simulink model "deadReckoning_VEX"  (R2017a)
settings: Solver=FixedStepAuto  StartTime=0.0  StopTime=inf  FixedStep=Ts  RelTol=1e-3  EnableMultiTasking=on
InitFcn:
  | robotParameters;
values from neighbouring files (symbols this model uses):
  ticksPerRot = 627.2    [robotParameters.m]
  Ts = 0.01    [robotParameters.m]
  wheelR = 0.052    [robotParameters.m]
undefined symbols (not defined in the file or in its folder): motorIp, motorSp
libraries: vexarmcortexlib x4, mobileRoboticsTrainingLib x1
settings Model: ExtModeTrigDuration=25  Creator=sseshadr  LastModifiedBy=shiremat
settings OptimizationCC: MaxStackSize=64
settings DebuggingCC: ParameterTunabilityLossMsg=error
settings HardwareCC: ProdBitPerPointer=32  ProdBitPerSizeT=32  ProdBitPerPtrDiffT=32  ProdLargestAtomicInteger=Long  ProdLargestAtomicFloat=Double  ProdWordSize=32  ProdHWDeviceType=ARM Compatible->ARM Cortex
settings SFSimCC: MATLABDynamicMemAlloc=off
settings RTWCC: SystemTargetFile=ert.tlc  HardwareBoard=ARM Cortex-based VEX Microcontroller  TLCOptions="-aInlineSetEventsForThisBaseRateFcn=TLC_FALSE -aSuppressMultiTaskScheduler=TLC_FALSE  -aRateBasedStepFcn=0"  TemplateMakefile=ert_default_tmf  Description=Embedded Coder  GenerateReport=on  Toolchain=GNU Tools for VEX ARM Cortex  IncludeHyperlinkInReport=on  LaunchReport=on  GenerateTraceInfo=on  GenerateTraceReport=on  GenerateTraceReportSl=on  GenerateTraceReportSf=on  GenerateTraceReportEml=on
settings CodeAppCC: ForceParamTrailComments=on  IgnoreCustomStorageClasses=off  OperatorAnnotations=on  SimulinkDataObjDesc=on  SFDataObjDesc=on  MATLABFcnDesc=on  InsertBlockDesc=on  MATLABSourceComments=on
settings ERTTargetCC: MultiwordLength=2048

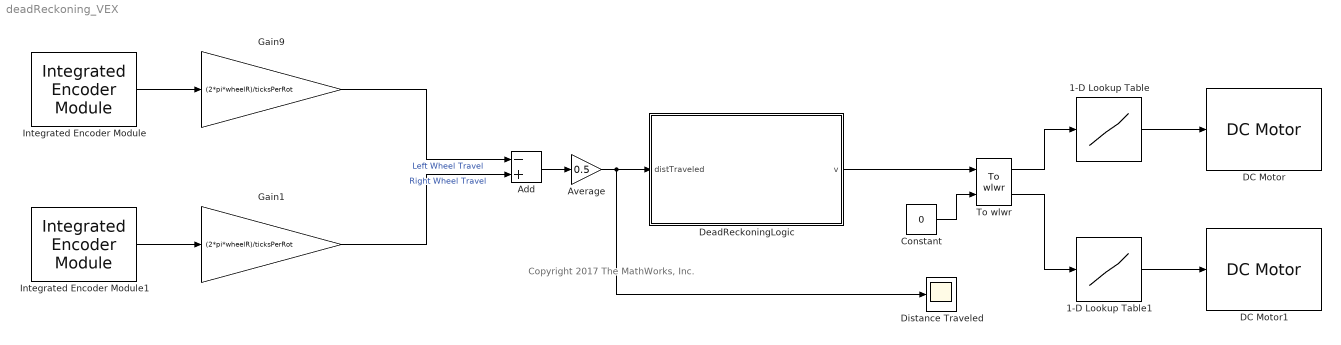
== system deadReckoning_VEX ==
  note: Copyright 2017 The MathWorks, Inc.
  1-D Lookup Table : Lookup_n-D  NumberOfTableDimensions=1  BreakpointsForDimension1=motorSp  Table=motorIp  ExtrapMethod=Clip  InternalRulePriority=Speed  RndMeth=Simplest  InputSameDT=on
  1-D Lookup Table1 : Lookup_n-D  NumberOfTableDimensions=1  BreakpointsForDimension1=motorSp  Table=motorIp  ExtrapMethod=Clip  InternalRulePriority=Speed  RndMeth=Simplest  InputSameDT=on
  Add : Sum  Inputs=-+
  Average : Gain  Gain=0.5
  Constant : Constant  Value=0
  DC Motor : vexarmcortexlib/Actuators/DC Motor  motor=10  scaleFactor=1/13.5  SimulationOut=off
      settings: SourceProductName=Simulink Coder Support Package for ARM Cortex-based VEX Microcontroller  SourceProductBaseCode=EC_VEX_MICRO
  DC Motor1 : vexarmcortexlib/Actuators/DC Motor  motor=1  scaleFactor=1/13.5  SimulationOut=off
      settings: SourceProductName=Simulink Coder Support Package for ARM Cortex-based VEX Microcontroller  SourceProductBaseCode=EC_VEX_MICRO
  DeadReckoningLogic : Stateflow chart  TreatAsAtomicUnit=on
  Distance Traveled : Scope
  Gain1 : Gain  Gain=(2*pi*wheelR)/ticksPerRot
  Gain9 : Gain  Gain=(2*pi*wheelR)/ticksPerRot
  Integrated Encoder Module : vexarmcortexlib/Sensors/Integrated Encoder Module  motorType=VEX 393 (High torque)  seqNumI2C=1  resetOption=No reset  rotVelocity=off  inputPortSim=off  SampleTime=Ts
      settings: SourceProductName=Simulink Coder Support Package for ARM Cortex-based VEX Microcontroller  SourceProductBaseCode=EC_VEX_MICRO
  Integrated Encoder Module1 : vexarmcortexlib/Sensors/Integrated Encoder Module  motorType=VEX 393 (High torque)  seqNumI2C=0  resetOption=No reset  rotVelocity=off  inputPortSim=off  SampleTime=Ts
      settings: SourceProductName=Simulink Coder Support Package for ARM Cortex-based VEX Microcontroller  SourceProductBaseCode=EC_VEX_MICRO
  To wlwr : mobileRoboticsTrainingLib/To wlwr  axleLength=axleLength  wheelR=wheelR
  wires:
  Average/1 -> DeadReckoningLogic/1(distTraveled), Distance Traveled/1
  DeadReckoningLogic/1(v) -> To wlwr/1
  Gain9/1 -> Add/1  "Left Wheel Travel"
  Add/1 -> Average/1
  Gain1/1 -> Add/2  "Right Wheel Travel"
  Constant/1 -> To wlwr/2
  To wlwr/1 -> 1-D Lookup Table/1
  To wlwr/2 -> 1-D Lookup Table1/1
  1-D Lookup Table/1 -> DC Motor/1
  1-D Lookup Table1/1 -> DC Motor1/1
  Integrated Encoder Module1/1 -> Gain1/1
  Integrated Encoder Module/1 -> Gain9/1

== stateflow chart deadReckoning_VEX/DeadReckoningLogic ==
  state MoveForward
    entry:
    v = 0.5;
  state Stop
    entry:
    v = 0;
  (default) -> MoveForward : %Start Dead Reckoning
  MoveForward -> Stop : [distTraveled > 1]
  data: v output; distTraveled input
